simulink model "CruiseControl_LogicIssue"  (R2015a)
settings: Solver=FixedStepDiscrete  StartTime=0.0  StopTime=2  FixedStep=0.1  RelTol=1e-3
PostLoadFcn:
  | CruiseControl_dd;
undefined symbols (not defined in the file or in its folder): holdrate, incdec, maxtspeed, mintspeed
settings Model: RecordCoverage=on  CovMetricSettings=dcme  CovHtmlReporting=off  covSaveCumulativeToWorkspaceVar=off  CovSaveSingleToWorkspaceVar=off  CovSFcnEnable=off  Creator=The MathWorks Inc.  LastModifiedBy=colosky
settings DataIOCC: SaveOutput=off  SaveTime=off
settings OptimizationCC: ConditionallyExecuteInputs=off  InlineParams=on  InlineInvariantSignals=on  ExpressionDepthLimit=2147483647  InitFltsAndDblsToZero=on  NoFixptDivByZeroProtection=on  OptimizeModelRefInitCode=on
settings DebuggingCC: SaveWithParameterizedLinksMsg=none  UnderspecifiedInitializationDetection=Classic  MergeDetectMultiDrivingBlocksExec=none  SolverPrmCheckMsg=warning  FcnCallInpInsideContextMsg=UseLocalSettings  StateNameClashWarn=warning  StrictBusMsg=ErrorOnBusTreatedAsVector
settings ModelReferenceCC: ModelReferenceNumInstancesAllowed=Single
settings SFSimCC: SimParseCustomCode=off
settings RTWCC: SystemTargetFile=ert.tlc  TemplateMakefile=ert_default_tmf  Description=Embedded Coder  GenerateReport=on  IncludeHyperlinkInReport=on  LaunchReport=on  PortableWordSizes=on  GenerateTraceInfo=on  GenerateTraceReport=on  GenerateTraceReportSl=on  GenerateTraceReportSf=on  GenerateTraceReportEml=on
settings CodeAppCC: IgnoreCustomStorageClasses=off  CustomSymbolStrGlobalVar=$N$M
settings ERTTargetCC: ParMdlRefBuildCompliant=on  CompOptLevelCompliant=on  ConcurrentExecutionCompliant=on  ERTFirstTimeCompliant=on  SupportContinuousTime=off  SupportVariableSizeSignals=off  ModelStepFunctionPrototypeControlCompliant=on  CPPClassGenCompliant=on  ERTCustomFileTemplate=example_file_process.tlc
settings ConfigComp: Description=Design Verifier Custom Configuration Component  DVMode=DesignErrorDetection  DVMaxProcessTime=3000  DVDisplayUnsatisfiableObjectives=on  DVAutomaticStubbing=off  DVMakeOutputFilesUnique=off  DVParameters=on  DVParametersUseConfig=on  DVModelCoverageObjectives=MCDC  DVMaxTestCaseSteps=500  DVTestSuiteOptimization=CombinedObjectives (Nonlinear Extended)  DVAssertions=EnableAll  DVProofAssumptions=EnableAll  DVIgnoreCovSatisfied=on  DVCoverageDataFile=cumcov_PartCvg.cvt  DVDetectIntegerOverflow=off  DVDetectDeadLogic=on  DVDetectActiveLogic=on  DVMaxViolationSteps=50  DVSaveDataFile=off  DVSaveHarnessModel=on  DVHarnessModelFileName=$ModelName$_harness_SLDV  DVModelReferenceHarness=on  DVReportIncludeGraphics=on  PSAutoStubLUT=off

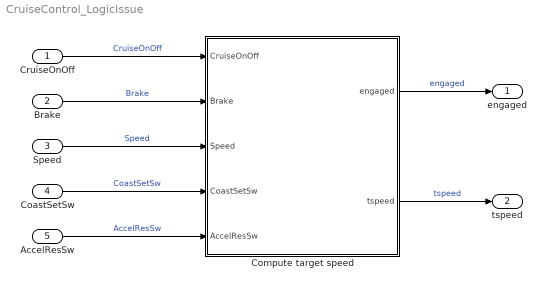
== system CruiseControl_LogicIssue ==
  CruiseOnOff : Inport  PortDimensions=1
  Brake : Inport  Port=2  PortDimensions=1
  Speed : Inport  Port=3  PortDimensions=1
  CoastSetSw : Inport  Port=4  PortDimensions=1
  AccelResSw : Inport  Port=5  PortDimensions=1
  Compute target speed : Stateflow chart  TreatAsAtomicUnit=on
  engaged : Outport
  tspeed : Outport  Port=2
  wires:
  AccelResSw/1 -> Compute target speed/5(AccelResSw)  "AccelResSw"
  Speed/1 -> Compute target speed/3(Speed)  "Speed"
  CoastSetSw/1 -> Compute target speed/4(CoastSetSw)  "CoastSetSw"
  CruiseOnOff/1 -> Compute target speed/1(CruiseOnOff)  "CruiseOnOff"
  Brake/1 -> Compute target speed/2(Brake)  "Brake"
  Compute target speed/1(engaged) -> engaged/1  "engaged"
  Compute target speed/2(tspeed) -> tspeed/1  "tspeed"

== stateflow chart CruiseControl_LogicIssue/Compute target speed ==
  state OFF
    en:
    engaged = false;
    tspeed = 0;
  state CRUISE
    state ON
      en: engaged = true;
      state Accel
        tspeed = tspeed + incdec;
      state Steady
      state Coast
        tspeed = tspeed - incdec;
      (junction 60) -> Accel
      (junction 57) -> (junction 60) : [after(10/holdrate...
          | *incdec,tick)]
      Accel -> (junction 57) [order 1]
      Steady -> Accel [order 1] : [hasChangedTo(AccelResSw,true) ...
          | && tspeed < maxtspeed]
      Accel -> Steady [order 2] : [!AccelResSw || ...
          | tspeed > maxtspeed]
      Steady -> (junction 75) [order 3] : [hasChangedTo(CoastSetSw,true)]
      (default) -> (junction 75)
      (junction 75) -> (junction 77) : {tspeed = Speed;}
      (junction 77) -> Steady
      Steady -> Coast [order 2] : [hasChangedTo(CoastSetSw,true) ...
          | && tspeed > mintspeed]
      Coast -> Steady [order 2] : [!CoastSetSw || ...
          | tspeed < mintspeed]
      (junction 72) -> Coast
      (junction 71) -> (junction 72) : [after(10/holdrate...
          | *incdec,tick)]
      Coast -> (junction 71) [order 1]
    state STANDBY
      en:
      engaged=false;
    (default) -> STANDBY
    ON -> STANDBY : [Brake||Speed> maxtspeed||Speed<mintspeed]
    STANDBY -> (junction 103) : [~Brake && ...
        | Speed<=maxtspeed && ...
        | Speed>=mintspeed]
    (junction 103) -> Steady [order 1] : [hasChangedTo(AccelResSw,true)...
        | &&tspeed!=0]
    (junction 103) -> (junction 106) [order 2]
    (junction 106) -> ON : [hasChangedTo(CoastSetSw,true)]
  (default) -> OFF
  OFF -> CRUISE : [CruiseOnOff]
  CRUISE -> OFF : [~CruiseOnOff]
  data: engaged output; CruiseOnOff input; Brake input; Speed input; CoastSetSw input; AccelResSw input; tspeed output; incdec parameter; holdrate parameter; maxtspeed parameter; mintspeed parameter
